simulink model "HydraulicPump_DigitalTwin"  (R2025b)
settings: Solver=VariableStepAuto  StartTime=0.0  StopTime=10.0  RelTol=1e-3
values from neighbouring files (symbols this model uses):
  faultGain = 2.5    [generate_data.m]
libraries: eeGeneralControl x1, dspstat3 x1
settings Model: LastModifiedBy=MSI

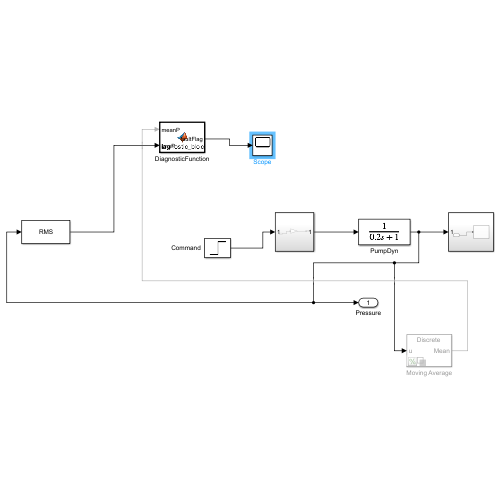
[thumbnail: Simulink's stored preview of the top-level diagram]
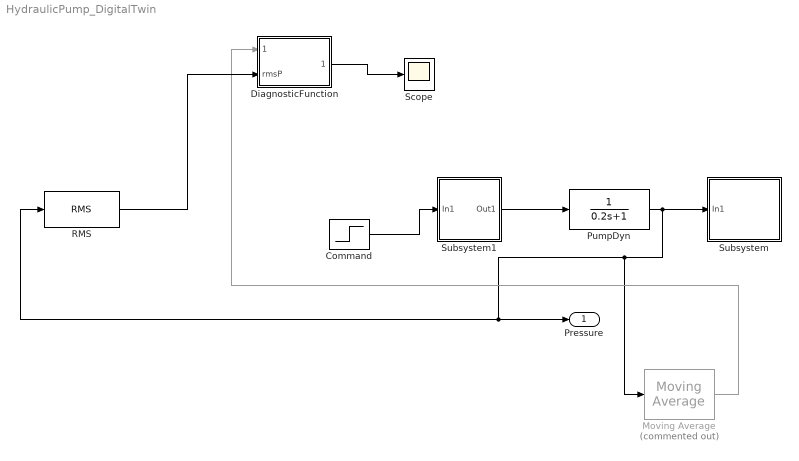
== system HydraulicPump_DigitalTwin ==
  Command : Step  Time=0  SampleTime=0
  DiagnosticFunction : MATLAB Function  TreatAsAtomicUnit=on  SystemSampleTime=0.1
  Moving Average : eeGeneralControl/Moving Average  Commented=on  VariantControl=Variant1  LabelModeActiveChoice=Discrete  f=1  x0=0  BufferSize=8192  Ts=0.1
      settings: LibrarySourceBlock=ee_sl_lib/General Control/Moving Average
  PumpDyn : TransferFcn  Denominator=[0.2 1]
  RMS : dspstat3/RMS  run=off  directionMode=Each column  dimension=1  InputProcessing=Columns as channels (frame based)  reset_popup=None
  Scope : Scope
      settings: ActiveDisplayYMinimum=-4.3990445149773478  ActiveDisplayYMaximum=5.5124508707593236
  Subsystem : Subsystem
  Subsystem1 : Subsystem
  Pressure : Outport
  wires:
  PumpDyn/1 -> Moving Average/1, RMS/1, Pressure/1, Subsystem/1(In1)
  Command/1 -> Subsystem1/1(In1)
  Subsystem1/1(Out1) -> PumpDyn/1
  Moving Average/1 -> DiagnosticFunction/1(meanP)
  RMS/1 -> DiagnosticFunction/2(rmsP)
  DiagnosticFunction/1(faultFlag) -> Scope/1

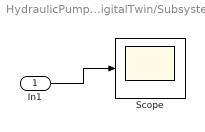
== system HydraulicPump_DigitalTwin/Subsystem ==
  In1 : Inport
  Scope : Scope
  wires:
  In1/1 -> Scope/1

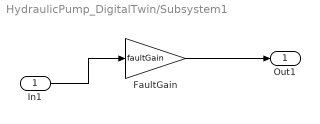
== system HydraulicPump_DigitalTwin/Subsystem1 ==
  In1 : Inport
  FaultGain : Gain  Gain=faultGain
  Out1 : Outport
  wires:
  In1/1 -> FaultGain/1
  FaultGain/1 -> Out1/1

== matlab function HydraulicPump_DigitalTwin/DiagnosticFunction ==
  data: meanP input; faultFlag output; rmsP input
function faultFlag = diagnostic_block(meanP, rmsP)
    %#codegen

    persistent mdl
    if isempty(mdl)
        mdl = loadLearnerForCoder('pumpMdlCompact');
    end

    X = table(meanP, rmsP, 'VariableNames', {'MeanPressure', 'RMSPressure'});
    faultLabel = predict(mdl, X);
    faultFlag = double(faultLabel); % 0 or 1
end
